simulink model "IPD"  (R2020a)
settings: Solver=VariableStepAuto  StartTime=0.0  StopTime=60  RelTol=1e-3
values from neighbouring files (symbols this model uses):
  Ac = [0, 1; -tf3.denominator{1}(3), -tf3.denominator{1}(2)]    [modelo.m]
  Bc = [0; tf3.numerator{1}(3)]    [modelo.m]
  Cc = [1, 0]    [modelo.m]
libraries: cstblocks x2
settings Model: Creator=jdavi  LastModifiedBy=jdavi

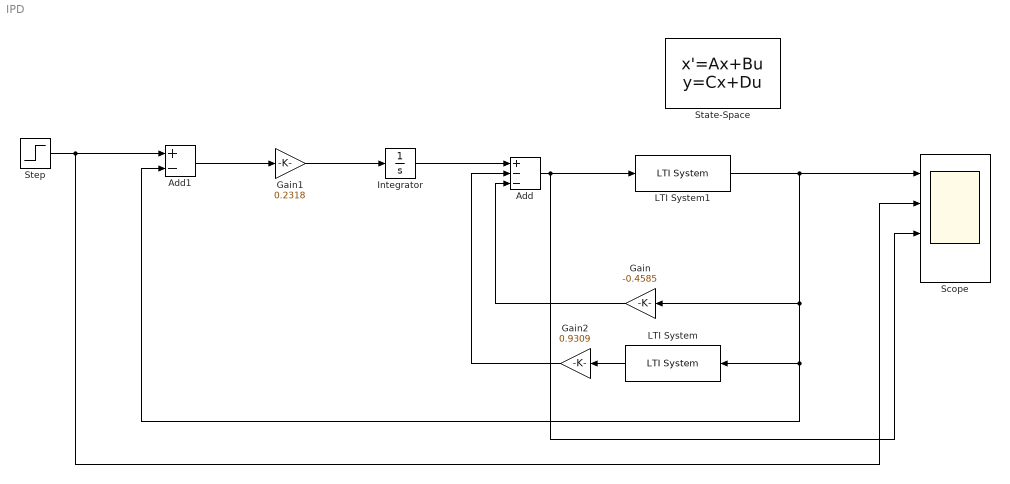
== system IPD ==
  Add : Sum  Inputs=+--
  Add1 : Sum  Inputs=+-
  Gain : Gain  Gain=-0.4585
  Gain1 : Gain  Gain=0.2318
  Gain2 : Gain  Gain=0.9309
  Integrator : Integrator
  LTI System : cstblocks/LTI System  sys=tf1  IC=[]
  LTI System1 : cstblocks/LTI System  sys=tf3  IC=[]
  Scope : Scope  NumInputPorts=4
  State-Space : StateSpace  A=Ac  B=Bc  C=Cc  D=0  InitialCondition=0
  Step : Step  Time=0  After=0.6  SampleTime=0
  wires:
  Add/1 -> Scope/3, LTI System1/1
  Gain1/1 -> Integrator/1
  Add1/1 -> Gain1/1
  Step/1 -> Scope/2, Add1/1
  Integrator/1 -> Add/1
  Gain/1 -> Add/3
  LTI System/1 -> Gain2/1
  Gain2/1 -> Add/2
  LTI System1/1 -> LTI System/1, Add1/2, Gain/1, Scope/1
